simulink model "detailed_model"  (R2020a)
settings: Solver=VariableStepAuto  StartTime=0.0  StopTime=3600  RelTol=1e-3
undefined symbols (not defined in the file): ee_sli_rtmsupport, gcbh
libraries: eeGeneralControl x6, eeGovernorG3 x1
settings Model: Creator=goria  LastModifiedBy=goria

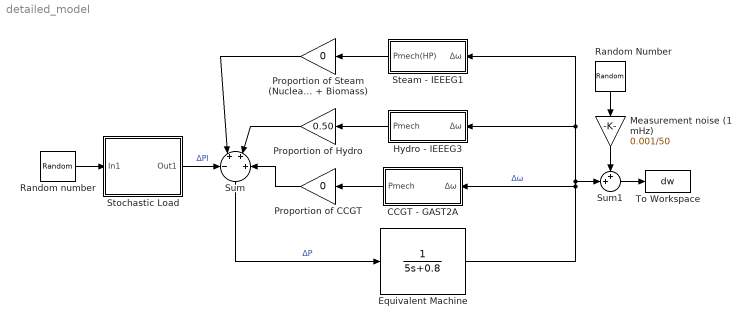
== system detailed_model ==
  CCGT - GAST2A : Subsystem
  Equivalent Machine : TransferFcn  Denominator=[5 0.8]
  Hydro - IEEEG3 : Subsystem
  Measurement noise (1 mHz) : Gain  Gain=0.001/50
  Proportion of CCGT : Gain  Gain=0
  Proportion of Hydro : Gain  Gain=0.50
  Proportion of Steam (Nuclear + Biomass) : Gain  Gain=0
  Random Number : RandomNumber  SampleTime=0.1
  Random number : RandomNumber  SampleTime=0.1
  Steam - IEEEG1 : Subsystem
  Stochastic Load : Subsystem
  Sum : Sum  Inputs=-+++
  Sum1 : Sum  Inputs=++|
  To Workspace : ToWorkspace  VariableName=dw  SaveFormat=Timeseries  SampleTime=1
  wires:
  Sum/1 -> Equivalent Machine/1  "ΔP"
  Random number/1 -> Stochastic Load/1(In1)
  Proportion of Steam (Nuclear + Biomass)/1 -> Sum/2
  Equivalent Machine/1 -> Steam - IEEEG1/1(Δω), Hydro - IEEEG3/1(Δω), Sum1/2, CCGT - GAST2A/1(Δω)  "Δω"
  Proportion of CCGT/1 -> Sum/4
  Proportion of Hydro/1 -> Sum/3
  Stochastic Load/1(Out1) -> Sum/1  "ΔPl"
  CCGT - GAST2A/1(Pmech) -> Proportion of CCGT/1
  Steam - IEEEG1/1(Pmech(HP)) -> Proportion of Steam (Nuclear + Biomass)/1
  Hydro - IEEEG3/1(Pmech) -> Proportion of Hydro/1
  Random Number/1 -> Measurement noise (1 mHz)/1
  Measurement noise (1 mHz)/1 -> Sum1/1
  Sum1/1 -> To Workspace/1

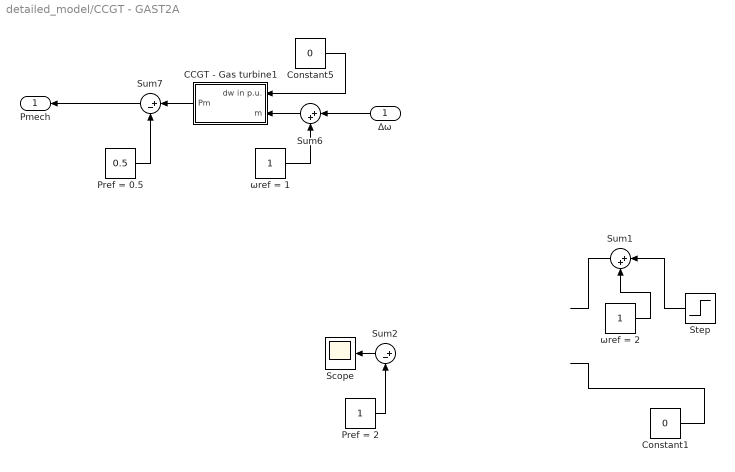
== system detailed_model/CCGT - GAST2A ==
  Δω : Inport
  CCGT - Gas turbine1 : Subsystem  mask(Gas Turbine Regulator){T0=0.5, Sbase=1, W=11, X=0.6, Y=1, Z=1, MAX=1.5, MIN=-0.13, a=1, b=0.05, c=1, Wmin=0.23, TF=0.4, KF=0, ECR=0.01, ETD=0.04, TCD=0.2, TR=950, TT=450, TI=0}
      mask prompts: T0 "Initial Output Power (T0, pu)"; Sbase "Rated Generator Power (S, MVA)"; W "Speed Governor Gain (W = 1/droop, pu MW/pu speed)"; X "Speed Governor Lead Constant (X, s)"; Y "Speed Governor Lag Constant (Y, s)"; Z "Speed Governor Mode (1 = droop, 0 = isochronus)"; MAX "Fuel Demand Signal Max Limit (MAX, pu)"; MIN "Fuel Demand Signal Min Limit (MIN, pu)"; a "Valve Positioner Parameter (a)"; b "Valve Positioner Time Constant (b, s)"; c "Valve Positioner Parameter (c)"; Wmin "No Load Fuel Consumption (Wmin)"; TF "Fuel System Time Constant (TF, s)"; KF "Fuel System External Feedback Loop Gain (KF)"; ECR "Delay of Combustion System (ECR, s)"; ETD "Transport Delay of Turbine and Exhaust System (ETD, s)"; TCD "Compressor Discharge Lag Time Contant (TCD, s)"; TR "Rated Exhaust Temperature (TR, degF)"; TT "Temperature Contoller Integration Constant (TT, degF)"; TI "Inertia (TI = 2*H)"
      mask help:
      | Full Rowen's model for HDGTs for dynamic studies.
      |
      | Limits of applicability:
      | 1. For simple cycle, single-shaft, generator drive only.
      | 2. Allowable speed range = 0.95 - 1.07 of rated speed.
      | 3. No heat recovery.
      | 4. ISO conditions.
      |
      | Model created according to the papers:
      | 1. W. I. Rowen,  Simplified mathematic representations of heavy-duty gas turbines, oct. 1983, p. 865
      | 2. Mohammad Reza Bank Tavakoli, Behrooz Vahidi and Wolfgang Gawlik, An Educational Guide to Extract
      | the Parameters of Heavy Duty Gas Turbines Model in Dynamic Studies Based on Operational Data
      mask Help:
      | Full Rowen's model for HDGTs for dynamic studies.
      | 
      | Limits of applicability:
      | 1. For simple cycle, single-shaft, generator drive only.
      | 2. Allowable speed range = 0.95 - 1.07 of rated speed.
      | 3. No heat recovery.
      | 4. ISO conditions.
      | 
      | Model created according to the papers:
      | 1. W. I. Rowen,  Simplified mathematic representations of heavy-duty gas turbines, oct. 1983, p. 865
      | 2. Mohammad Reza Bank Tavakoli, Behrooz Vahidi and Wolfgang Gawlik, An Educational Guide to Extract
      | the Parameters of Heavy Duty Gas Turbines Model in Dynamic Studies Based on Operational Data
  Constant1 : Constant  Value=0
  Constant5 : Constant  Value=0
  Pref = 0.5 : Constant  Value=0.5
  Pref = 2 : Constant
  Scope : Scope
  Step : Step  After=+0.01  SampleTime=0
  Sum1 : Sum  Inputs=|++
  Sum2 : Sum  Inputs=|+-
  Sum6 : Sum  Inputs=|++
  Sum7 : Sum  Inputs=|+-
  ωref = 1 : Constant
  ωref = 2 : Constant
  Pmech : Outport
  wires:
  Pref = 0.5/1 -> Sum7/2
  CCGT - Gas turbine1/1(Pm) -> Sum7/1
  ωref = 1/1 -> Sum6/2
  Sum7/1 -> Pmech/1
  Sum6/1 -> CCGT - Gas turbine1/2(m)
  Δω/1 -> Sum6/1
  Constant5/1 -> CCGT - Gas turbine1/1(dw in p.u.)
  Step/1 -> Sum1/1
  ωref = 2/1 -> Sum1/2
  ? -> Sum2/1
  Sum2/1 -> Scope/1
  Pref = 2/1 -> Sum2/2
  Sum1/1 -> ?
  Constant1/1 -> ?

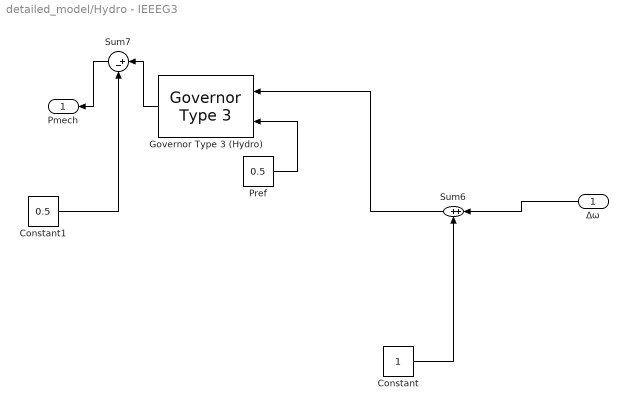
== system detailed_model/Hydro - IEEEG3 ==
  Δω : Inport
  Constant : Constant
  Constant1 : Constant  Value=0.5
  Governor Type 3 (Hydro) : eeGovernorG3/Governor Type 3  pu_speed_reference=1  pu_torque0=0.5  Ts=-1  T_g=0.52  T_p=0.07  U_o=0.15  U_c=-0.15  P_max=1  P_min=-1  R_perm=0.05  R_temp=0.6  T_r=25  T_w=5  a_11=0.75  a_13=0.75  a_21=0.75  a_23=0.75
      settings: SourceProductBaseCode=PS
  Pref : Constant  Value=0.5
  Sum6 : Sum  Inputs=|++
  Sum7 : Sum  Inputs=|+-
  Pmech : Outport
  wires:
  Pref/1 -> Governor Type 3 (Hydro)/2
  Constant/1 -> Sum6/2
  Δω/1 -> Sum6/1
  Sum6/1 -> Governor Type 3 (Hydro)/1
  Sum7/1 -> Pmech/1
  Governor Type 3 (Hydro)/1 -> Sum7/1
  Constant1/1 -> Sum7/2

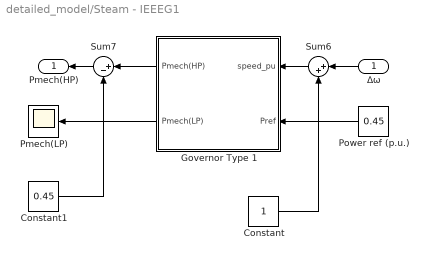
== system detailed_model/Steam - IEEEG1 ==
  Δω : Inport
  Constant : Constant
  Constant1 : Constant  Value=0.45
  Governor Type 1 : Subsystem  AncestorBlock=eeGovernorG1/Governor Type 1  LoadFcn=ee_sli_rtmsupport( 'loadfcn', gcbh );  mask(Governor Type 1){pu_speed_reference=1, pu_torque0=0.45, Ts=-1, K=11, T_1=0.2, T_2=0, T_3=0.1, U_o=0.1, U_c=-0.1, P_max=0.98, P_min=0, T_4=0.25, K_1=0.22, K_2=0, T_5=4, K_3=0.22, K_4=0, T_6=4, K_5=0.3, K_6=0, T_7=0.4, K_7=0.26, K_8=0, db1=0.036/50}
      mask prompts: pu_speed_reference "physmod:ee:library:comments:control:eeGovernorG1:SpeedReferencepu_MP"; pu_torque0 "physmod:ee:library:comments:control:eeGovernorG1:InitialTorquepu_MP"; Ts "physmod:ee:library:comments:control:eeGovernorG1:SampleTime1ForInherited_MP"; K "physmod:ee:library:comments:control:eeGovernorG1:GovernorGain1droopKpu_MP"; T_1 "physmod:ee:library:comments:control:eeGovernorG1:LagTimeConstantT_1s_MP"; T_2 "physmod:ee:library:comments:control:eeGovernorG1:LeadTimeConstantT_2s_MP"; T_3 "physmod:ee:library:comments:control:eeGovernorG1:ValvePositionTimeConstantT_3s_MP"; U_o "physmod:ee:library:comments:control:eeGovernorG1:MaximumValveOpeningRateU_opus_MP"; U_c "physmod:ee:library:comments:control:eeGovernorG1:MaximumValveClosingRateU_cpus_MP"; P_max "physmod:ee:library:comments:control:eeGovernorG1:MaximumValveOpeningOnMWCapabilityP_maxpu_MP"; P_min "physmod:ee:library:comments:control:eeGovernorG1:MinimumValveOpeningOnMWCapabilityP_minpu_MP"; T_4 "physmod:ee:library:comments:control:eeGovernorG1:TimeConstantForSteamInletT_4s_MP"; K_1 "physmod:ee:library:comments:control:eeGovernorG1:HPFractionK_1_MP"; K_2 "physmod:ee:library:comments:control:eeGovernorG1:LPFractionK2_MP"; T_5 "physmod:ee:library:comments:control:eeGovernorG1:TimeConstantForSecondBoilerPassT_5s_MP"; K_3 "physmod:ee:library:comments:control:eeGovernorG1:HPFractionK_3_MP"; K_4 "physmod:ee:library:comments:control:eeGovernorG1:LPFractionK_4_MP"; T_6 "physmod:ee:library:comments:control:eeGovernorG1:TimeConstantForThirdBoilerPassT_6s_MP"; K_5 "physmod:ee:library:comments:control:eeGovernorG1:HPFractionK_5_MP"; K_6 "physmod:ee:library:comments:control:eeGovernorG1:LPFractionK_6_MP"; T_7 "physmod:ee:library:comments:control:eeGovernorG1:TimeConstantForFourthBoilerPassT_7s_MP"; K_7 "physmod:ee:library:comments:control:eeGovernorG1:HPFractionK_7_MP"; K_8 "physmod:ee:library:comments:control:eeGovernorG1:LPFractionK_8_MP"; db1 "physmod:ee:library:comments:control:eeGovernorG1:Deadband_MP"
      mask help: physmod:ee:library:comments:control:eeGovernorG1:GovernorType1_MD
      mask init:
      | timeDomain = ee.mask.getTimeDomain(Ts);
      settings: CopyFcn=ee_sli_rtmsupport( 'copyfcn', gcbh );  DeleteFcn=ee_sli_rtmsupport( 'deletefcn', gcbh );  ModelCloseFcn=ee_sli_rtmsupport( 'modelclosefcn', gcbh );  PostSaveFcn=ee_sli_rtmsupport( 'postsavefcn', gcbh );  PreCopyFcn=ee_sli_rtmsupport( 'precopyfcn', gcbh );  OpenFcn=ee_sli_rtmsupport( 'openfcn', gcbh );  CloseFcn=ee_sli_rtmsupport( 'closefcn', gcbh );  PreDeleteFcn=ee_sli_rtmsupport( 'predeletefcn', gcbh );
      mask Help: web(nesl_help(gcbh))
      mask TypeOptions Ts:
      | Lead-Lag/Ts | Low-Pass Filter/Ts | Low-Pass Filter1/Ts | Low-Pass Filter2/Ts | Low-Pass Filter3/Ts | Integrator
      | (Discrete or Continuous)/Ts
      mask DialogControl TabGeneral Prompt: physmod:ee:library:comments:control:eeGovernorG1:tab_General
      mask DialogControl pu_speed_reference Prompt: Speed reference (pu)
      mask DialogControl pu_torque0 Prompt: Initial torque (pu)
      mask DialogControl Ts Prompt: Sample time (-1 for inherited)
      mask DialogControl TabGovernor Prompt: physmod:ee:library:comments:control:eeGovernorG1:tab_Governor
      mask DialogControl K Prompt: Governor gain (1/droop), K (pu)
      mask DialogControl T_1 Prompt: Lag time constant, T_1 (s)
      mask DialogControl T_2 Prompt: Lead time constant, T_2 (s)
      mask DialogControl T_3 Prompt: Valve position time constant, T_3 (s)
      mask DialogControl U_o Prompt: Maximum valve opening rate, U_o (pu/s)
      mask DialogControl U_c Prompt: Maximum valve closing rate, U_c (pu/s)
      mask DialogControl P_max Prompt: Maximum valve opening, on MW capability, P_max (pu)
      mask DialogControl P_min Prompt: Minimum valve opening, on MW capability, P_min (pu)
      mask DialogControl T_4 Prompt: Time constant for steam inlet, T_4 (s)
      mask DialogControl K_1 Prompt: HP fraction, K_1
      mask DialogControl K_2 Prompt: LP fraction, K2
      mask DialogControl T_5 Prompt: Time constant for second boiler pass, T_5 (s)
      mask DialogControl K_3 Prompt: HP fraction, K_3
      mask DialogControl K_4 Prompt: LP fraction, K_4
      mask DialogControl T_6 Prompt: Time constant for third boiler pass, T_6 (s)
      mask DialogControl K_5 Prompt: HP fraction, K_5
      mask DialogControl K_6 Prompt: LP fraction, K_6
      mask DialogControl T_7 Prompt: Time constant for fourth boiler pass, T_7 (s)
      mask DialogControl K_7 Prompt: HP fraction, K_7
      mask DialogControl K_8 Prompt: LP fraction, K_8
      mask DialogControl db1 Prompt: Deadband
      mask Display: ee.mask.drawGovernors(gcb);
  Pmech(LP) : Scope
  Power ref (p.u.) : Constant  Value=0.45
  Sum6 : Sum  Inputs=|++
  Sum7 : Sum  Inputs=|+-
  Pmech(HP) : Outport
  wires:
  Power ref (p.u.)/1 -> Governor Type 1/2(Pref)
  Governor Type 1/2(Pmech(LP)) -> Pmech(LP)/1
  Δω/1 -> Sum6/1
  Sum6/1 -> Governor Type 1/1(speed_pu)
  Constant/1 -> Sum6/2
  Governor Type 1/1(Pmech(HP)) -> Sum7/1
  Sum7/1 -> Pmech(HP)/1
  Constant1/1 -> Sum7/2

== system detailed_model/Stochastic Load ==
  In1 : Inport
  Gain : Gain  Gain=sqrt(2*6e-6)*100
  Transfer Fcn : TransferFcn  Denominator=[0 1]
  Out1 : Outport
  wires:
  In1/1 -> Gain/1
  Gain/1 -> Transfer Fcn/1
  Transfer Fcn/1 -> Out1/1

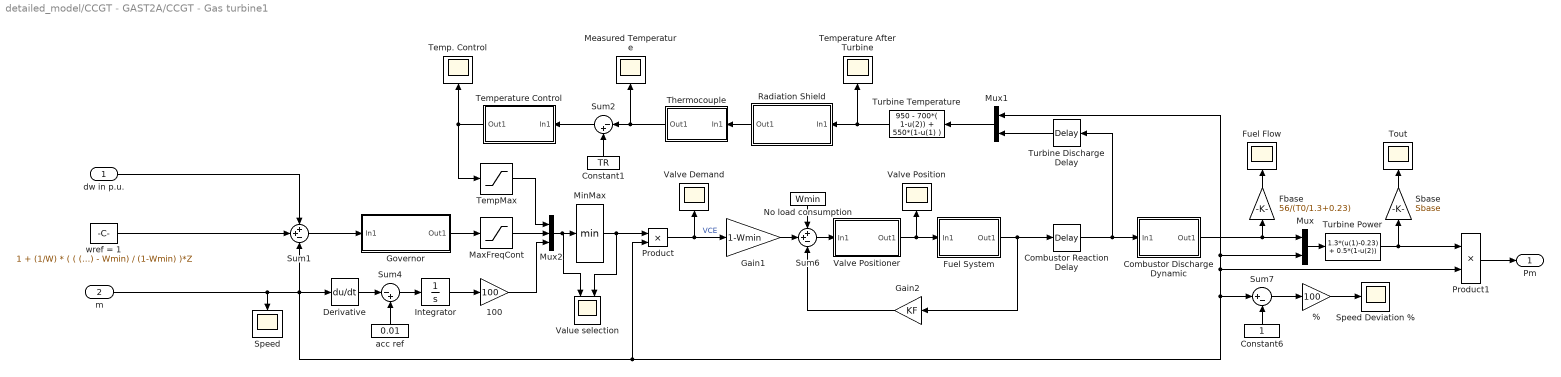
== system detailed_model/CCGT - GAST2A/CCGT - Gas turbine1 ==
  dw in p.u. : Inport
  m : Inport  Port=2
  % : Gain  Gain=100
  100 : Gain  Gain=100
  Combustor Discharge Dynamic : Subsystem
      mask Display: fprintf('1/(TCD.s+1)')
  Combustor Reaction Delay : TransportDelay  DelayTime=ECR  InitialOutput=T0/1.3+0.23
  Constant1 : Constant  Value=TR
  Constant6 : Constant
  Derivative : Derivative
  Fbase : Gain  Gain=56/(T0/1.3+0.23)
  Fuel Flow : Scope
  Fuel System : Subsystem
      mask Display: fprintf('1/(TF.s+1)')
  Gain1 : Gain  Gain=1-Wmin
  Gain2 : Gain  Gain=KF
  Governor : Subsystem
      mask Display: fprintf('W(Xs+1)/(Ys+Z)')
  Integrator : Integrator  InitialCondition=1
  MaxFreqCont : Saturate  UpperLimit=MAX  LowerLimit=MIN
  Measured Temperature : Scope
  MinMax : MinMax
  Mux : Mux  Inputs=2
  Mux1 : Mux  Inputs=2
  Mux2 : Mux  Inputs=3
  No load consumption : Constant  Value=Wmin
  Product : Product  RndMeth=Zero
  Product1 : Product  RndMeth=Zero
  Radiation Shield : Subsystem
      mask Display: fprintf('0.2/(15s+1)+0.8')
  Sbase : Gain  Gain=Sbase
  Speed : Scope
  Speed Deviation % : Scope
  Sum1 : Sum  Inputs=++-
  Sum2 : Sum  Inputs=|-+
  Sum4 : Sum  Inputs=|-+
  Sum6 : Sum  Inputs=++-
  Sum7 : Sum  Inputs=|+-
  Temp. Control : Scope
  TempMax : Saturate  UpperLimit=MAX  LowerLimit=MIN
  Temperature After Turbine : Scope
  Temperature Control : Subsystem
      mask Display: fprintf('(3.3s+1)/TT.s')
  Thermocouple : Subsystem
      mask Display: fprintf('1/(2.5s+1)')
  Tout : Scope
  Turbine Discharge Delay : TransportDelay  DelayTime=ETD  InitialOutput=T0/1.3+0.23
  Turbine Power : Fcn  Expr=1.3*(u(1)-0.23) + 0.5*(1-u(2))
  Turbine Temperature : Fcn  Expr=950 - 700*( 1-u(2)) + 550*(1-u(1) )
  Value selection : Scope  NumInputPorts=2
  Valve Demand : Scope
  Valve Position : Scope
  Valve Positioner : Subsystem
      mask Display: fprintf('a/(b.s+c)')
  acc ref : Constant  Value=0.01
  wref = 1 : Constant  Value=1 + (1/W) * ( ( (T0/1.3 + 0.23)*(c/a) - Wmin) / (1-Wmin) )*Z
  Pm : Outport
  wires:
  m/1 -> Sum1/3, Derivative/1, Product1/2, Mux1/1, Mux/2, Sum7/1, Product/2, Speed/1
  Sum1/1 -> Governor/1(In1)
  Thermocouple/1(Out1) -> Sum2/1, Measured Temperature/1
  Constant1/1 -> Sum2/2
  Integrator/1 -> 100/1
  Sum4/1 -> Integrator/1
  Derivative/1 -> Sum4/1
  acc ref/1 -> Sum4/2
  Combustor Discharge Dynamic/1(Out1) -> Mux/1, Fbase/1
  Turbine Power/1 -> Product1/1, Sbase/1
  Product/1 -> Valve Demand/1, Gain1/1  "VCE"
  Sum6/1 -> Valve Positioner/1(In1)
  Sum2/1 -> Temperature Control/1(In1)
  Valve Positioner/1(Out1) -> Fuel System/1(In1), Valve Position/1
  Fuel System/1(Out1) -> Gain2/1, Combustor Reaction Delay/1
  Combustor Reaction Delay/1 -> Combustor Discharge Dynamic/1(In1), Turbine Discharge Delay/1
  Gain2/1 -> Sum6/3
  Turbine Discharge Delay/1 -> Mux1/2
  Gain1/1 -> Sum6/2
  No load consumption/1 -> Sum6/1
  Temperature Control/1(Out1) -> Temp. Control/1, TempMax/1
  Mux/1 -> Turbine Power/1
  Governor/1(Out1) -> MaxFreqCont/1
  Constant6/1 -> Sum7/2
  Sum7/1 -> %/1
  %/1 -> Speed Deviation %/1
  Turbine Temperature/1 -> Radiation Shield/1(In1), Temperature After Turbine/1
  Mux1/1 -> Turbine Temperature/1
  Radiation Shield/1(Out1) -> Thermocouple/1(In1)
  Sbase/1 -> Tout/1
  Fbase/1 -> Fuel Flow/1
  Product1/1 -> Pm/1
  MinMax/1 -> Product/1, Value selection/2
  Mux2/1 -> Value selection/1, MinMax/1
  MaxFreqCont/1 -> Mux2/2
  100/1 -> Mux2/3
  TempMax/1 -> Mux2/1
  wref = 1/1 -> Sum1/2
  dw in p.u./1 -> Sum1/1

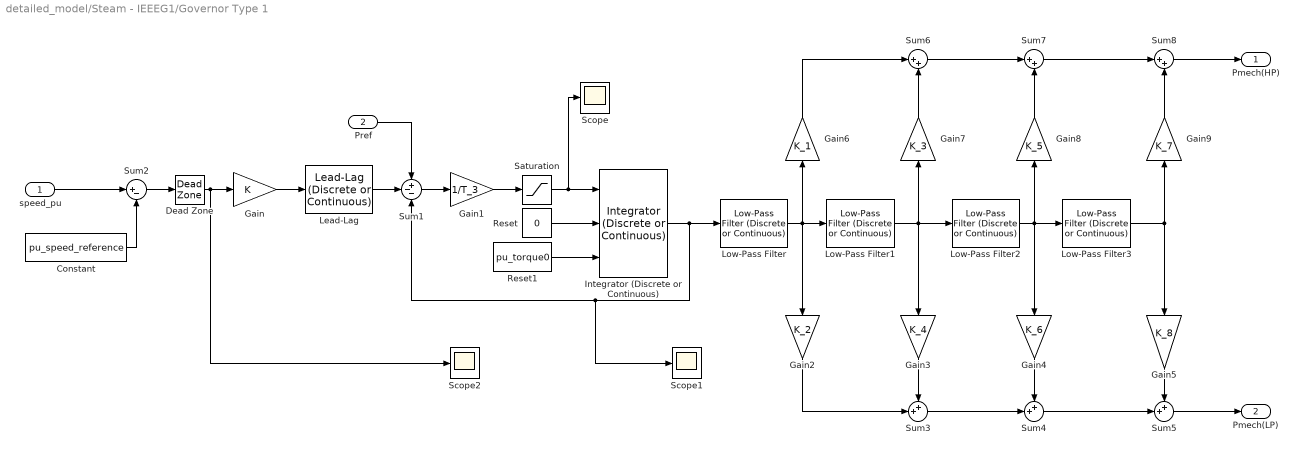
== system detailed_model/Steam - IEEEG1/Governor Type 1 ==
  speed_pu : Inport  SampleTime=Ts
  Pref : Inport  Port=2  SampleTime=Ts
  Constant : Constant  Value=pu_speed_reference
  Dead Zone : DeadZone  LowerValue=-db1  UpperValue=db1  ZeroCross=off  SaturateOnIntegerOverflow=on
  Gain : Gain  Gain=K
  Gain1 : Gain  Gain=1/T_3
  Gain2 : Gain  Gain=K_2
  Gain3 : Gain  Gain=K_4
  Gain4 : Gain  Gain=K_6
  Gain5 : Gain  Gain=K_8
  Gain6 : Gain  Gain=K_1
  Gain7 : Gain  Gain=K_3
  Gain8 : Gain  Gain=K_5
  Gain9 : Gain  Gain=K_7
  Integrator (Discrete or Continuous) : eeGeneralControl/Integrator (Discrete or Continuous)  LabelModeActiveChoice=Discrete  ExternalReset=level  LimitType=Anti-windup  B=P_max  A=P_min  Ts=Ts
      settings: SourceProductBaseCode=PS
  Lead-Lag : eeGeneralControl/Lead-Lag (Discrete or Continuous)  T1=T_2  T2=T_1  B=inf  A=-inf  init_option=Inherited from block input  x0=0  Ts=Ts
      settings: SourceProductBaseCode=PS
  Low-Pass Filter : eeGeneralControl/Low-Pass Filter (Discrete or Continuous)  K=1  T=T_4  B=inf  A=-inf  init_option=Inherited from block input  x0=0  Ts=Ts
  Low-Pass Filter1 : eeGeneralControl/Low-Pass Filter (Discrete or Continuous)  K=1  T=T_5  B=inf  A=-inf  init_option=Inherited from block input  x0=0  Ts=Ts
  Low-Pass Filter2 : eeGeneralControl/Low-Pass Filter (Discrete or Continuous)  K=1  T=T_6  B=inf  A=-inf  init_option=Inherited from block input  x0=0  Ts=Ts
  Low-Pass Filter3 : eeGeneralControl/Low-Pass Filter (Discrete or Continuous)  K=1  T=T_7  B=inf  A=-inf  init_option=Inherited from block input  x0=0  Ts=Ts
  Reset : Constant  Value=0
  Reset1 : Constant  Value=pu_torque0
  Saturation : Saturate  UpperLimit=U_o  LowerLimit=U_c
  Scope : Scope
  Scope1 : Scope
  Scope2 : Scope
  Sum1 : Sum  Inputs=+--
  Sum2 : Sum  Inputs=|+-
  Sum3 : Sum  Inputs=++|
  Sum4 : Sum  Inputs=++|
  Sum5 : Sum  Inputs=++|
  Sum6 : Sum  Inputs=|++
  Sum7 : Sum  Inputs=|++
  Sum8 : Sum  Inputs=|++
  Pmech(HP) : Outport  VectorParamsAs1DForOutWhenUnconnected=off
  Pmech(LP) : Outport  Port=2  VectorParamsAs1DForOutWhenUnconnected=off
  wires:
  speed_pu/1 -> Sum2/1
  Constant/1 -> Sum2/2
  Sum2/1 -> Dead Zone/1
  Gain/1 -> Lead-Lag/1
  Lead-Lag/1 -> Sum1/2
  Integrator (Discrete or Continuous)/1 -> Sum1/3, Scope1/1, Low-Pass Filter/1
  Pref/1 -> Sum1/1
  Gain1/1 -> Saturation/1
  Saturation/1 -> Scope/1, Integrator (Discrete or Continuous)/1
  Reset/1 -> Integrator (Discrete or Continuous)/2
  Low-Pass Filter/1 -> Gain6/1, Low-Pass Filter1/1, Gain2/1
  Low-Pass Filter2/1 -> Gain8/1, Gain4/1, Low-Pass Filter3/1
  Low-Pass Filter1/1 -> Gain7/1, Gain3/1, Low-Pass Filter2/1
  Low-Pass Filter3/1 -> Gain5/1, Gain9/1
  Gain6/1 -> Sum6/1
  Gain7/1 -> Sum6/2
  Gain3/1 -> Sum3/1
  Gain2/1 -> Sum3/2
  Gain4/1 -> Sum4/1
  Sum3/1 -> Sum4/2
  Sum4/1 -> Sum5/2
  Gain5/1 -> Sum5/1
  Gain8/1 -> Sum7/2
  Sum6/1 -> Sum7/1
  Gain9/1 -> Sum8/2
  Sum7/1 -> Sum8/1
  Sum8/1 -> Pmech(HP)/1
  Sum5/1 -> Pmech(LP)/1
  Reset1/1 -> Integrator (Discrete or Continuous)/3
  Sum1/1 -> Gain1/1
  Dead Zone/1 -> Scope2/1, Gain/1

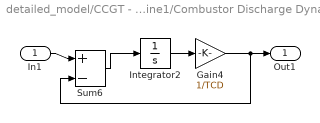
== system detailed_model/CCGT - GAST2A/CCGT - Gas turbine1/Combustor Discharge Dynamic ==
  In1 : Inport
  Gain4 : Gain  Gain=1/TCD
  Integrator2 : Integrator  InitialCondition=TCD*(T0/1.3+0.23)
  Sum6 : Sum  Inputs=|+-
  Out1 : Outport
  wires:
  Integrator2/1 -> Gain4/1
  Gain4/1 -> Sum6/2, Out1/1
  Sum6/1 -> Integrator2/1
  In1/1 -> Sum6/1

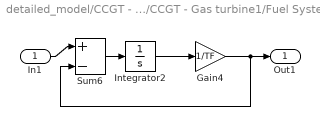
== system detailed_model/CCGT - GAST2A/CCGT - Gas turbine1/Fuel System ==
  In1 : Inport
  Gain4 : Gain  Gain=1/TF
  Integrator2 : Integrator  InitialCondition=TF*(T0/1.3+0.23)
  Sum6 : Sum  Inputs=|+-
  Out1 : Outport
  wires:
  Integrator2/1 -> Gain4/1
  Gain4/1 -> Sum6/2, Out1/1
  Sum6/1 -> Integrator2/1
  In1/1 -> Sum6/1

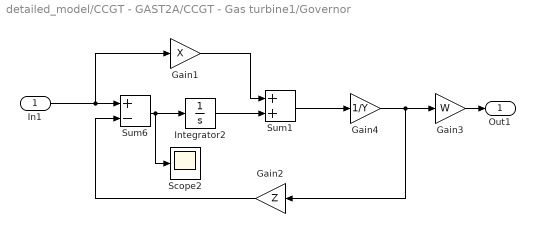
== system detailed_model/CCGT - GAST2A/CCGT - Gas turbine1/Governor ==
  In1 : Inport
  Gain1 : Gain  Gain=X
  Gain2 : Gain  Gain=Z
  Gain3 : Gain  Gain=W
  Gain4 : Gain  Gain=1/Y
  Integrator2 : Integrator  InitialCondition=(Y-Z*X)*(1/W)*(((T0/1.3+0.23)*(c/a)-Wmin)/(1-Wmin))
  Scope2 : Scope
  Sum1 : Sum
  Sum6 : Sum  Inputs=+-
  Out1 : Outport
  wires:
  Gain4/1 -> Gain2/1, Gain3/1
  Sum6/1 -> Scope2/1, Integrator2/1
  In1/1 -> Sum6/1, Gain1/1
  Integrator2/1 -> Sum1/2
  Gain1/1 -> Sum1/1
  Gain2/1 -> Sum6/2
  Sum1/1 -> Gain4/1
  Gain3/1 -> Out1/1

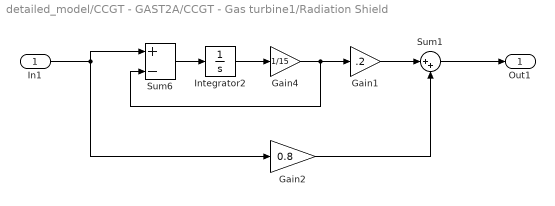
== system detailed_model/CCGT - GAST2A/CCGT - Gas turbine1/Radiation Shield ==
  In1 : Inport
  Gain1 : Gain  Gain=.2
  Gain2 : Gain  Gain=0.8
  Gain4 : Gain  Gain=1/15
  Integrator2 : Integrator  InitialCondition=15*(950-700*(1-T0/1.3-0.23))
  Sum1 : Sum  Inputs=|++
  Sum6 : Sum  Inputs=|+-
  Out1 : Outport
  wires:
  Integrator2/1 -> Gain4/1
  Gain4/1 -> Sum6/2, Gain1/1
  Sum6/1 -> Integrator2/1
  In1/1 -> Sum6/1, Gain2/1
  Gain1/1 -> Sum1/1
  Sum1/1 -> Out1/1
  Gain2/1 -> Sum1/2

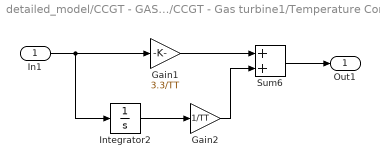
== system detailed_model/CCGT - GAST2A/CCGT - Gas turbine1/Temperature Control ==
  In1 : Inport
  Gain1 : Gain  Gain=3.3/TT
  Gain2 : Gain  Gain=1/TT
  Integrator2 : Integrator  InitialCondition=950
  Sum6 : Sum
  Out1 : Outport
  wires:
  Sum6/1 -> Out1/1
  In1/1 -> Gain1/1, Integrator2/1
  Gain1/1 -> Sum6/1
  Integrator2/1 -> Gain2/1
  Gain2/1 -> Sum6/2

== system detailed_model/CCGT - GAST2A/CCGT - Gas turbine1/Thermocouple ==
  In1 : Inport
  Gain4 : Gain  Gain=1/2.5
  Integrator2 : Integrator  InitialCondition=2.5*((950-700*(1-T0/1.3-0.23)))
  Sum6 : Sum  Inputs=|+-
  Out1 : Outport
  wires:
  Integrator2/1 -> Gain4/1
  Gain4/1 -> Sum6/2, Out1/1
  Sum6/1 -> Integrator2/1
  In1/1 -> Sum6/1

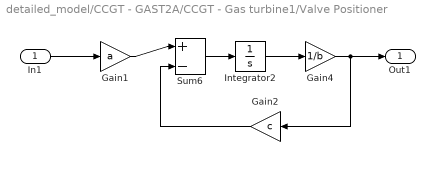
== system detailed_model/CCGT - GAST2A/CCGT - Gas turbine1/Valve Positioner ==
  In1 : Inport
  Gain1 : Gain  Gain=a
  Gain2 : Gain  Gain=c
  Gain4 : Gain  Gain=1/b
  Integrator2 : Integrator  InitialCondition=b*(T0/1.3+0.23)
  Sum6 : Sum  Inputs=|+-
  Out1 : Outport
  wires:
  Integrator2/1 -> Gain4/1
  Gain4/1 -> Out1/1, Gain2/1
  Sum6/1 -> Integrator2/1
  In1/1 -> Gain1/1
  Gain1/1 -> Sum6/1
  Gain2/1 -> Sum6/2
